simulink model "sl_subsys_trig4"  (Simulink 6.0)
settings: Solver=FixedStepDiscrete  SolverMode=SingleTasking  StartTime=0.0  StopTime=10.0  RelTol=1e-3
settings Model: CovMetricSettings=d  Creator=The MathWorks Inc.  LastModifiedBy=batserve  ExtModeAutoUpdateStatusClock=off
settings OptimizationCC: BlockReduction=off  BooleanDataType=off
settings DebuggingCC: CheckExecutionContextPreStartOutputMsg=on  CheckExecutionContextRuntimeOutputMsg=on  SolverPrmCheckMsg=none
settings HardwareCC: TargetUnknown=on

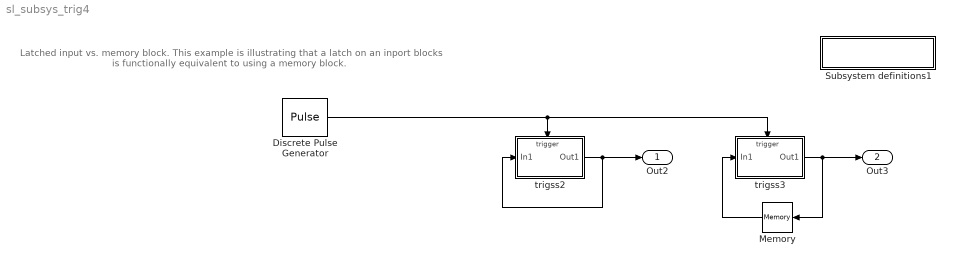
== system sl_subsys_trig4 ==
  note: Latched input vs. memory block.
      |
      | This example is illustrating that a latch on an inport blocks is
      | functionally equivalent to using a memory block.
  " Subsystem definitions1" : Subsystem  PropExecContextAcrossSSBoundary=on
      settings: OpenFcn=helpview([matlabroot,'/toolbox/simulink/simdemos/sl_subsys_definitions.html']);
      mask Display: disp('Subsystem\ndefinitions')
  Discrete Pulse Generator : DiscretePulseGenerator
  Memory : Memory  Orientation=left  InheritSampleTime=on
  trigss2 : Subsystem  TreatAsAtomicUnit=on  PropExecContextAcrossSSBoundary=on
  trigss3 : Subsystem  TreatAsAtomicUnit=on  PropExecContextAcrossSSBoundary=on
  Out2 : Outport
  Out3 : Outport  Port=2
  wires:
  trigss2/1(Out1) -> Out2/1, trigss2/1(In1)
  trigss3/1(Out1) -> Out3/1, Memory/1
  Memory/1 -> trigss3/1(In1)
  Discrete Pulse Generator/1 -> trigss2/Trigger, trigss3/Trigger

== system sl_subsys_trig4/ Subsystem definitions1 ==

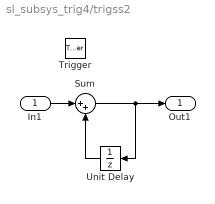
== system sl_subsys_trig4/trigss2 ==
  In1 : Inport  Port=1  LatchInput=on
  Trigger : TriggerPort
  Sum : Sum  Inputs=|++  SaturateOnIntegerOverflow=on  InputSameDT=on
  Unit Delay : UnitDelay  Orientation=left  X0=1  SampleTime=-1
  Out1 : Outport
  wires:
  In1/1 -> Sum/1
  Sum/1 -> Unit Delay/1, Out1/1
  Unit Delay/1 -> Sum/2

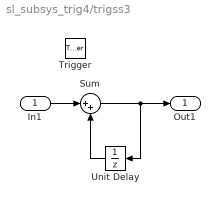
== system sl_subsys_trig4/trigss3 ==
  In1 : Inport  Port=1  LatchInput=off
  Trigger : TriggerPort
  Sum : Sum  Inputs=|++  SaturateOnIntegerOverflow=on  InputSameDT=on
  Unit Delay : UnitDelay  Orientation=left  X0=1  SampleTime=-1
  Out1 : Outport
  wires:
  In1/1 -> Sum/1
  Sum/1 -> Out1/1, Unit Delay/1
  Unit Delay/1 -> Sum/2
